simulink subsystem "MotoSimpleEngine"  (R2024a)
settings: Solver=VariableStepAuto  StartTime=0.0  StopTime=10.0  RelTol=1e-3
libraries: autolibsharedcommon x1, autolibpowerinfoutils x1, autolibsharedmappedengines x1
settings Model: ModifiedByFormat=The MathWorks, Inc.  Creator=The MathWorks, Inc.  LastModifiedBy=The MathWorks, Inc.
settings RTWCC: GPUComputeCapability=3.5

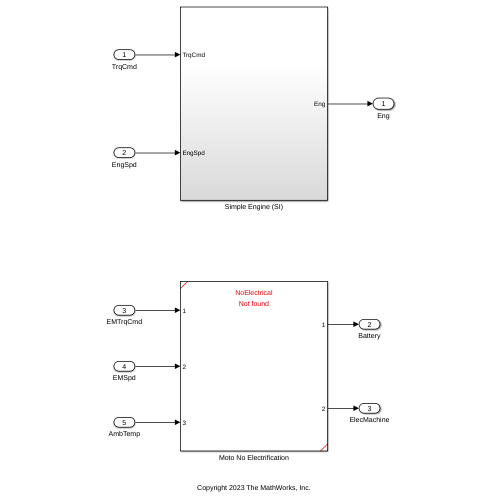
[thumbnail: Simulink's stored preview of the top-level diagram]
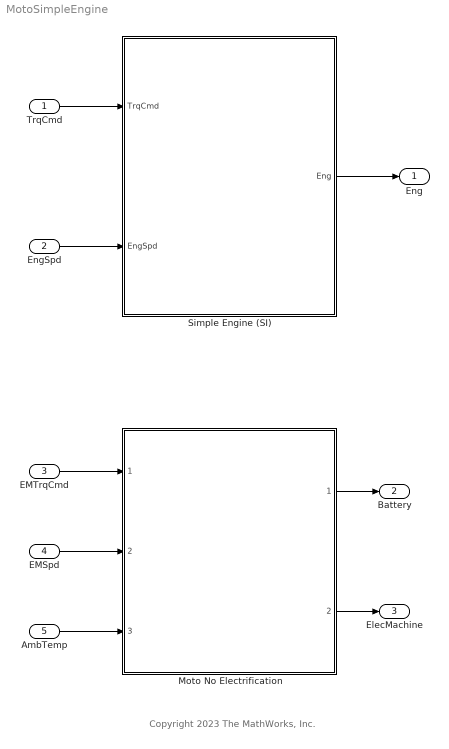
== system MotoSimpleEngine ==
  note: Copyright 2023 The MathWorks, Inc.
  TrqCmd : Inport
  EngSpd : Inport  Port=2
  EMTrqCmd : Inport  Port=3
  EMSpd : Inport  Port=4
  AmbTemp : Inport  Port=5
  Moto No Electrification : Subsystem  VariantControl=Moto No Electrification  ReferencedSubsystem=NoElectrical
  Simple Engine (SI) : Subsystem  VariantControl=Simple Engine (SI)
  Eng : Outport
  Battery : Outport  Port=2
  ElecMachine : Outport  Port=3
  wires:
  TrqCmd/1 -> Simple Engine (SI)/1(TrqCmd)
  EngSpd/1 -> Simple Engine (SI)/2(EngSpd)
  Simple Engine (SI)/1(Eng) -> Eng/1
  AmbTemp/1 -> Moto No Electrification/3
  EMSpd/1 -> Moto No Electrification/2
  EMTrqCmd/1 -> Moto No Electrification/1
  Moto No Electrification/2 -> ElecMachine/1
  Moto No Electrification/1 -> Battery/1

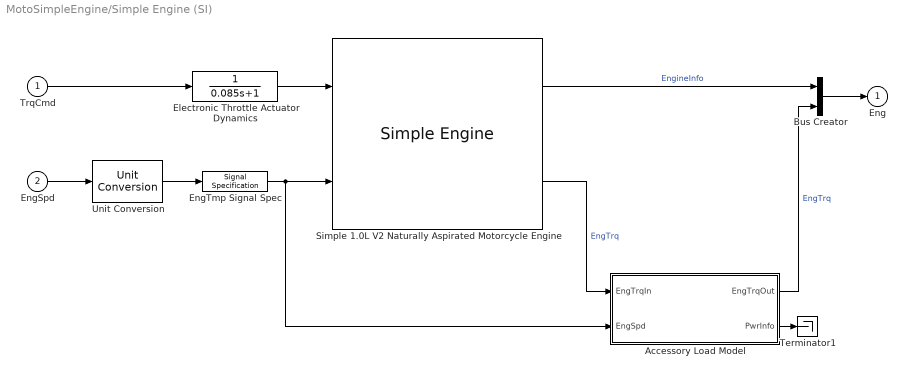
== system MotoSimpleEngine/Simple Engine (SI) ==
  TrqCmd : Inport
  EngSpd : Inport  Port=2
  Accessory Load Model : Subsystem
  Bus Creator : BusCreator  Inputs=2
  Electronic Throttle Actuator Dynamics : TransferFcn  Denominator=[0.085 1]
  EngTmp Signal Spec : SignalSpecification  Unit=rpm
  Simple 1.0L V2 Naturally Aspirated Motorcycle Engine : autolibsharedmappedengines/Simple Engine  f_tqmax=PlntEngTqMax  f_tqmax_n_bpt=PlntEngTqMaxBpt  Lhv=PlntEngLhv  Sg=PlntEngSg  BsfcAvg=PlntEngBsfcAvg  aMode=6
  Terminator1 : Terminator
  Unit Conversion : UnitConversion
  Eng : Outport
  wires:
  Accessory Load Model/1(EngTrqOut) -> Bus Creator/2  "EngTrq"
  Bus Creator/1 -> Eng/1
  Accessory Load Model/2(PwrInfo) -> Terminator1/1
  Electronic Throttle Actuator Dynamics/1 -> Simple 1.0L V2 Naturally Aspirated Motorcycle Engine/1
  Simple 1.0L V2 Naturally Aspirated Motorcycle Engine/2 -> Accessory Load Model/1(EngTrqIn)  "EngTrq"
  Unit Conversion/1 -> EngTmp Signal Spec/1
  EngTmp Signal Spec/1 -> Accessory Load Model/2(EngSpd), Simple 1.0L V2 Naturally Aspirated Motorcycle Engine/2
  Simple 1.0L V2 Naturally Aspirated Motorcycle Engine/1 -> Bus Creator/1  "EngineInfo"
  TrqCmd/1 -> Electronic Throttle Actuator Dynamics/1
  EngSpd/1 -> Unit Conversion/1

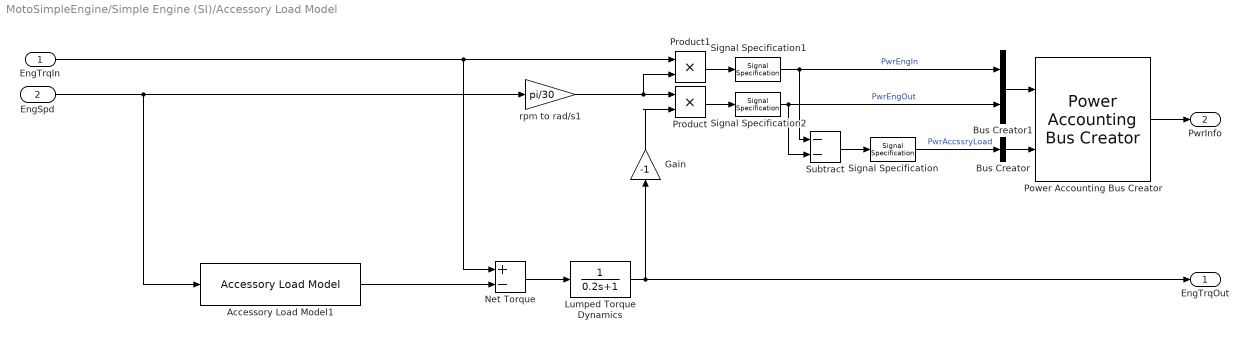
== system MotoSimpleEngine/Simple Engine (SI)/Accessory Load Model ==
  EngTrqIn : Inport
  EngSpd : Inport  Port=2
  Accessory Load Model1 : autolibsharedcommon/Accessory Load Model  AccPwrTbl=PlntEngAccPwrTbl  AccSpdBpts=PlntEngAccSpdBpt  aMode=aMode
  Bus Creator : BusCreator  Inputs=1
  Bus Creator1 : BusCreator  Inputs=2
  Gain : Gain  Gain=-1
  Lumped Torque Dynamics : TransferFcn  Denominator=[0.2 1]
  Net Torque : Sum  Inputs=+-
  Power Accounting Bus Creator : autolibpowerinfoutils/Power Accounting Bus Creator  AssctBlkSelPopup=Parent  RefBlkName='libraryname/blkname'  PwrTrnsfrdCheckBox=on  PwrNotTrnsfrdCheckBox=on  PwrStoredCheckBox=off  aMode=6
  Product : Product
  Product1 : Product
  Signal Specification : SignalSpecification  Unit=W
  Signal Specification1 : SignalSpecification  Unit=W
  Signal Specification2 : SignalSpecification  Unit=W
  Subtract : Sum  Inputs=--
  rpm to rad/s1 : Gain  Gain=pi/30
  EngTrqOut : Outport  Unit=N*m  VectorParamsAs1DForOutWhenUnconnected=off
  PwrInfo : Outport  Port=2  VectorParamsAs1DForOutWhenUnconnected=off
  wires:
  Accessory Load Model1/1 -> Net Torque/2
  EngSpd/1 -> rpm to rad/s1/1, Accessory Load Model1/1
  Lumped Torque Dynamics/1 -> EngTrqOut/1, Gain/1
  Net Torque/1 -> Lumped Torque Dynamics/1
  Bus Creator/1 -> Power Accounting Bus Creator/2
  Bus Creator1/1 -> Power Accounting Bus Creator/1
  EngTrqIn/1 -> Product1/1, Net Torque/1
  Subtract/1 -> Signal Specification/1
  Signal Specification/1 -> Bus Creator/1  "PwrAccssryLoad"
  Power Accounting Bus Creator/1 -> PwrInfo/1
  Product/1 -> Signal Specification2/1
  Product1/1 -> Signal Specification1/1
  rpm to rad/s1/1 -> Product1/2, Product/1
  Signal Specification1/1 -> Subtract/1, Bus Creator1/1  "PwrEngIn"
  Signal Specification2/1 -> Subtract/2, Bus Creator1/2  "PwrEngOut"
  Gain/1 -> Product/2
